simulink model "SecRwRtStBkReclnIsPosChk"  (R2024b)
settings: Solver=FixedStepDiscrete  StartTime=0.0  StopTime=10.0  FixedStep=0.01  RelTol=1e-3
undefined symbols (not defined in the file or in its folder): KeSMSuSecRwStBackPosDelta_Val, KeSMSuSecRwStBackPosTolr_Val, KeSMSuVehicleModelConfig_Val
libraries: StIsPosChkLib x19, simulink x8
(part 1 of 2)
settings Model: Creator=sn2xws  LastModifiedBy=sn55gm
settings Model: ModifiedHistory=|
  | 2023.8.1 V2.0.0 CR421790 增加模式21-26
  | 2024.3.14
  | V2.3.0
  | Bug 813950 童锁Lock，Mode1_Easy Entry Mode 不应调用失败
  | 2024.5.7 V3.0.0 557 eze模式变更
  | 2024.7.8 V3.0.1 557模式流程V1.9
  | 2024.8.15 V3.0.2 智享模式需要计算目标位置，不能直接判断到位置，posalready赋值0
  | 2024.8.20 V3.0.3 MD32到位置不看二排靠背
  | 2024.9.5 V3.0.4 增加Md56，注释掉不用的模式
  | 2024.10.14 V3.0.5 增加Md57，Md58
  | 2024.10.29 V3.0.6 6s版本不使用md8目标位置
  | 2024.11.5 V3.0.7 6s版本不动Md32
  | 2024.11.27 V3.0.8 Md57 运行时二排不能直接判断到位置
  | 2024.12.18 V3.0.8 md53 到位置不应看二排靠背，md32，md53同时动时，应用较小目标位置
  | 25.5.20 V3.12.0 童锁Md56应报成功
  | 25.7.1 V3.13.0 新增Md61 Md62
settings SolverCC: AlgebraicLoopSolver=TrustRegion
settings DataIOCC: SaveFormat=StructureWithTime  ReturnWorkspaceOutputs=off
settings OptimizationCC: DefaultParameterBehavior=Inlined  EnhancedBackFolding=on  PassReuseOutputArgsAs=Individual arguments  ZeroExternalMemoryAtStartup=off  ZeroInternalMemoryAtStartup=off  OptimizeBlockOrder=speed  DifferentSizesBufferReuse=on  OptimizationCustomize=off  EfficientTunableParamExpr=on
settings DebuggingCC: ParameterTunabilityLossMsg=error  UnconnectedInputMsg=warning  UnconnectedOutputMsg=warning  UnconnectedLineMsg=warning  ArithmeticOperatorsInVariantConditions=warning
settings ModelReferenceCC: EnableRefExpFcnMdlSchedulingChecks=on  ModelReferenceNumInstancesAllowed=Single
settings SFSimCC: MATLABDynamicMemAlloc=off  CustomCodeUndefinedFunction=UseInterfaceOnly
settings RTWCC: Description=AUTOSAR  SystemTargetFile=autosar.tlc  GenCodeOnly=on  TemplateMakefile=ert_default_tmf  GenerateReport=on  IncludeHyperlinkInReport=on  LaunchReport=on  DataTypeReplacement=CDataTypesFixedWidth  GenerateTraceInfo=on  GenerateTraceReport=on  GenerateTraceReportSl=on  GenerateTraceReportSf=on  GenerateTraceReportEml=on  GPUComputeCapability=3.5
settings CodeAppCC: ForceParamTrailComments=on  IgnoreCustomStorageClasses=off  OperatorAnnotations=on  SimulinkDataObjDesc=on  SFDataObjDesc=on  InsertBlockDesc=on
settings STFCustomTargetCC: TargetLangStandard=C99 (ISO)  MultiwordLength=256  ParMdlRefBuildCompliant=on  CompOptLevelCompliant=on  IncludeMdlTerminateFcn=off  CombineOutputUpdateFcns=on  SuppressErrorStatus=on  ERTCustomFileBanners=on  SupportNonFinite=off  SupportComplex=off  SupportContinuousTime=off  SupportNonInlinedSFcns=off  RemoveResetFunc=on  MATLABClassNameForMDSCustomization=Simulink.SoftwareTarget.ERTCustomization  AutosarCompliant=on  UseToolchainInfoCompliant=on  LookupTableObjectStructAxisOrder=2,1,3,4,...  LUTObjectStructOrderEvenSpacing=Size,Table,Breakpoints  SystemTargetFile=autosar.tlc
settings ERTTargetCC: TargetLangStandard=C99 (ISO)  ConcurrentExecutionCompliant=off  IncludeMdlTerminateFcn=off  SuppressErrorStatus=on  SupportNonFinite=off  SupportComplex=off  ModelStepFunctionPrototypeControlCompliant=off  CPPClassGenCompliant=off  AutosarCompliant=on  LookupTableObjectStructAxisOrder=2,1,3,4,...  LUTObjectStructOrderEvenSpacing=Size,Table,Breakpoints  ERTCustomFileTemplate=example_file_process.tlc  ERTFilePackagingFormat=Compact  BooleanTrueId=TRUE  BooleanFalseId=FALSE  DynamicArrayContainerType=coder::array

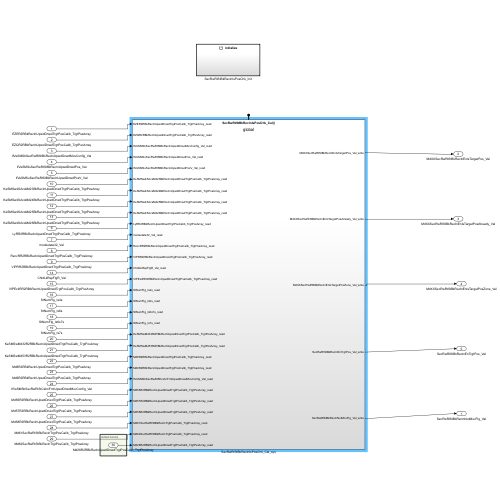
[thumbnail: Simulink's stored preview of the top-level diagram]
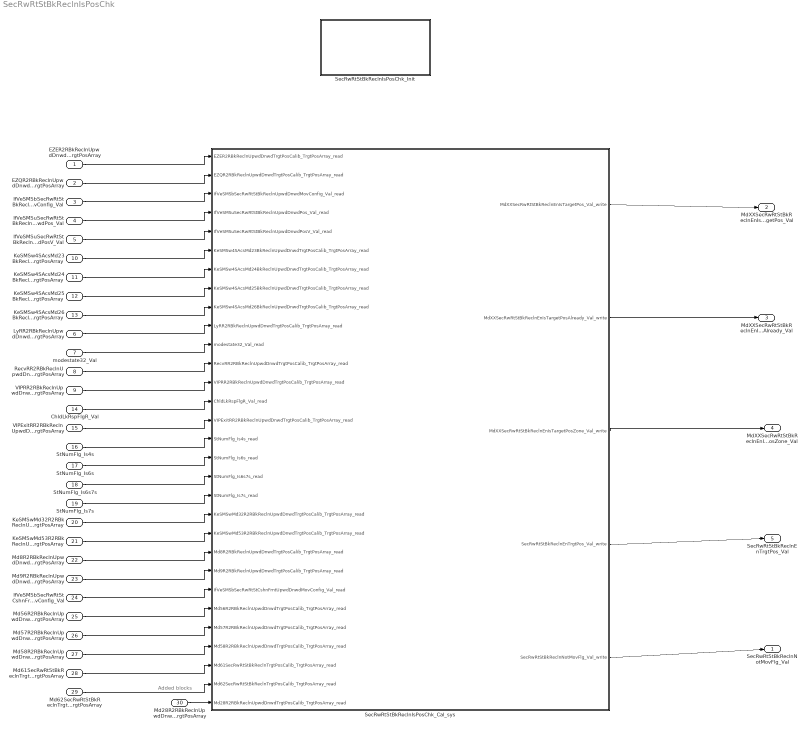
== system SecRwRtStBkReclnIsPosChk ==
  note: Added blocks
  EZER2RBkReclnUpwdDnwdTrgtPosCalib_TrgtPosArray : Inport  Description=|  OutDataTypeStr=uint16  PortDimensions=3
      | 0:Pos
      | 1:Max
      | 2:Min
  EZQR2RBkReclnUpwdDnwdTrgtPosCalib_TrgtPosArray : Inport  Description=|  Port=2  OutDataTypeStr=uint16  PortDimensions=3
      | 0:Pos
      | 1:Max
      | 2:Min
  IfVeSMSbSecRwRtStBkReclnUpwdDnwdMovConfig_Val : Inport  Port=3  OutDataTypeStr=boolean  PortDimensions=1
  IfVeSMSuSecRwRtStBkReclnUpwdDnwdPos_Val : Inport  Port=4  OutDataTypeStr=uint16  PortDimensions=1
  IfVeSMSuSecRwRtStBkReclnUpwdDnwdPosV_Val : Inport  Port=5  OutDataTypeStr=boolean  PortDimensions=1
  LyRR2RBkReclnUpwdDnwdTrgtPosCalib_TrgtPosArray : Inport  Description=|  Port=6  OutDataTypeStr=uint16  PortDimensions=3
      | 0:Pos
      | 1:Max
      | 2:Min
  modestate32_Val : Inport  Port=7  OutDataTypeStr=uint32  PortDimensions=1
  RecvRR2RBkReclnUpwdDnwdTrgtPosCalib_TrgtPosArray : Inport  Description=|  Port=8  OutDataTypeStr=uint16  PortDimensions=3
      | 0:Pos
      | 1:Max
      | 2:Min
  VIPRR2RBkReclnUpwdDnwdTrgtPosCalib_TrgtPosArray : Inport  Description=|  Port=9  OutDataTypeStr=uint16  PortDimensions=3
      | 0:Pos
      | 1:Max
      | 2:Min
  KeSMSw4SAcsMd23BkReclnUpwdDnwdTrgtPosCalib_TrgtPosArray : Inport  Description=|  Port=10  OutDataTypeStr=uint16  PortDimensions=3
      | 0:Pos
      | 1:Max
      | 2:Min
  KeSMSw4SAcsMd24BkReclnUpwdDnwdTrgtPosCalib_TrgtPosArray : Inport  Description=|  Port=11  OutDataTypeStr=uint16  PortDimensions=3
      | 0:Pos
      | 1:Max
      | 2:Min
  KeSMSw4SAcsMd25BkReclnUpwdDnwdTrgtPosCalib_TrgtPosArray : Inport  Description=|  Port=12  OutDataTypeStr=uint16  PortDimensions=3
      | 0:Pos
      | 1:Max
      | 2:Min
  KeSMSw4SAcsMd26BkReclnUpwdDnwdTrgtPosCalib_TrgtPosArray : Inport  Description=|  Port=13  OutDataTypeStr=uint16  PortDimensions=3
      | 0:Pos
      | 1:Max
      | 2:Min
  ChldLkRspFlgR_Val : Inport  Port=14  OutDataTypeStr=boolean  PortDimensions=1
  VIPExitRR2RBkReclnUpwdDnwdTrgtPosCalib_TrgtPosArray : Inport  Description=|  Port=15  OutDataTypeStr=uint16  PortDimensions=3
      | 0:Pos
      | 1:Max
      | 2:Min
  StNumFlg_Is4s : Inport  Port=16  OutDataTypeStr=boolean  PortDimensions=1
  StNumFlg_Is6s : Inport  Port=17  OutDataTypeStr=boolean  PortDimensions=1
  StNumFlg_Is6s7s : Inport  Port=18  OutDataTypeStr=boolean  PortDimensions=1
  StNumFlg_Is7s : Inport  Port=19  OutDataTypeStr=boolean  PortDimensions=1
  KeSMSwMd32R2RBkReclnUpwdDnwdTrgtPosCalib_TrgtPosArray : Inport  Description=|  Port=20  OutDataTypeStr=uint16  PortDimensions=3
      | 0:Pos
      | 1:Max
      | 2:Min
  KeSMSwMd53R2RBkReclnUpwdDnwdTrgtPosCalib_TrgtPosArray : Inport  Description=|  Port=21  OutDataTypeStr=uint16  PortDimensions=3
      | 0:Pos
      | 1:Max
      | 2:Min
  Md8R2RBkReclnUpwdDnwdTrgtPosCalib_TrgtPosArray : Inport  Description=|  Port=22  OutDataTypeStr=uint16  PortDimensions=3
      | 0:Pos
      | 1:Max
      | 2:Min
  Md9R2RBkReclnUpwdDnwdTrgtPosCalib_TrgtPosArray : Inport  Description=|  Port=23  OutDataTypeStr=uint16  PortDimensions=3
      | 0:Pos
      | 1:Max
      | 2:Min
  IfVeSMSbSecRwRtStCshnFrntUpwdDnwdMovConfig_Val : Inport  Port=24  OutDataTypeStr=boolean  PortDimensions=1
  Md56R2RBkReclnUpwdDnwdTrgtPosCalib_TrgtPosArray : Inport  Description=|  Port=25  OutDataTypeStr=uint16  PortDimensions=3
      | 0:Pos
      | 1:Max
      | 2:Min
  Md57R2RBkReclnUpwdDnwdTrgtPosCalib_TrgtPosArray : Inport  Description=|  Port=26  OutDataTypeStr=uint16  PortDimensions=3
      | 0:Pos
      | 1:Max
      | 2:Min
  Md58R2RBkReclnUpwdDnwdTrgtPosCalib_TrgtPosArray : Inport  Description=|  Port=27  OutDataTypeStr=uint16  PortDimensions=3
      | 0:Pos
      | 1:Max
      | 2:Min
  Md61SecRwRtStBkReclnTrgtPosCalib_TrgtPosArray : Inport  Description=|  Port=28  OutDataTypeStr=uint16  PortDimensions=3
      | 0:Pos
      | 1:Max
      | 2:Min
  Md62SecRwRtStBkReclnTrgtPosCalib_TrgtPosArray : Inport  Description=|  Port=29  OutDataTypeStr=uint16  PortDimensions=3
      | 0:Pos
      | 1:Max
      | 2:Min
  Md28R2RBkReclnUpwdDnwdTrgtPosCalib_TrgtPosArray : Inport  Description=|  Port=30  OutDataTypeStr=uint16  PortDimensions=3
      | 0:Pos
      | 1:Max
      | 2:Min
  SecRwRtStBkReclnIsPosChk_Cal_sys : Subsystem
  SecRwRtStBkReclnIsPosChk_Init : Subsystem
  SecRwRtStBkReclnNotMovFlg_Val : Outport  OutDataTypeStr=boolean  PortDimensions=1  VectorParamsAs1DForOutWhenUnconnected=off
  MdXXSecRwRtStBkReclnEnIsTargetPos_Val : Outport  Port=2  OutDataTypeStr=uint32  PortDimensions=1  VectorParamsAs1DForOutWhenUnconnected=off
  MdXXSecRwRtStBkReclnEnIsTargetPosAlready_Val : Outport  Port=3  OutDataTypeStr=uint32  PortDimensions=1  VectorParamsAs1DForOutWhenUnconnected=off
  MdXXSecRwRtStBkReclnEnIsTargetPosZone_Val : Outport  Port=4  OutDataTypeStr=uint32  PortDimensions=1  VectorParamsAs1DForOutWhenUnconnected=off
  SecRwRtStBkReclnEnTrgtPos_Val : Outport  Port=5  OutDataTypeStr=uint16  PortDimensions=1  VectorParamsAs1DForOutWhenUnconnected=off
  wires:
  EZER2RBkReclnUpwdDnwdTrgtPosCalib_TrgtPosArray/1 -> SecRwRtStBkReclnIsPosChk_Cal_sys/1(EZER2RBkReclnUpwdDnwdTrgtPosCalib_TrgtPosArray_read)
  EZQR2RBkReclnUpwdDnwdTrgtPosCalib_TrgtPosArray/1 -> SecRwRtStBkReclnIsPosChk_Cal_sys/2(EZQR2RBkReclnUpwdDnwdTrgtPosCalib_TrgtPosArray_read)
  IfVeSMSbSecRwRtStBkReclnUpwdDnwdMovConfig_Val/1 -> SecRwRtStBkReclnIsPosChk_Cal_sys/3(IfVeSMSbSecRwRtStBkReclnUpwdDnwdMovConfig_Val_read)
  IfVeSMSuSecRwRtStBkReclnUpwdDnwdPos_Val/1 -> SecRwRtStBkReclnIsPosChk_Cal_sys/4(IfVeSMSuSecRwRtStBkReclnUpwdDnwdPos_Val_read)
  IfVeSMSuSecRwRtStBkReclnUpwdDnwdPosV_Val/1 -> SecRwRtStBkReclnIsPosChk_Cal_sys/5(IfVeSMSuSecRwRtStBkReclnUpwdDnwdPosV_Val_read)
  LyRR2RBkReclnUpwdDnwdTrgtPosCalib_TrgtPosArray/1 -> SecRwRtStBkReclnIsPosChk_Cal_sys/10(LyRR2RBkReclnUpwdDnwdTrgtPosCalib_TrgtPosArray_read)
  modestate32_Val/1 -> SecRwRtStBkReclnIsPosChk_Cal_sys/11(modestate32_Val_read)
  RecvRR2RBkReclnUpwdDnwdTrgtPosCalib_TrgtPosArray/1 -> SecRwRtStBkReclnIsPosChk_Cal_sys/12(RecvRR2RBkReclnUpwdDnwdTrgtPosCalib_TrgtPosArray_read)
  VIPRR2RBkReclnUpwdDnwdTrgtPosCalib_TrgtPosArray/1 -> SecRwRtStBkReclnIsPosChk_Cal_sys/13(VIPRR2RBkReclnUpwdDnwdTrgtPosCalib_TrgtPosArray_read)
  SecRwRtStBkReclnIsPosChk_Cal_sys/1(MdXXSecRwRtStBkReclnEnIsTargetPos_Val_write) -> MdXXSecRwRtStBkReclnEnIsTargetPos_Val/1
  SecRwRtStBkReclnIsPosChk_Cal_sys/2(MdXXSecRwRtStBkReclnEnIsTargetPosAlready_Val_write) -> MdXXSecRwRtStBkReclnEnIsTargetPosAlready_Val/1
  SecRwRtStBkReclnIsPosChk_Cal_sys/3(MdXXSecRwRtStBkReclnEnIsTargetPosZone_Val_write) -> MdXXSecRwRtStBkReclnEnIsTargetPosZone_Val/1
  SecRwRtStBkReclnIsPosChk_Cal_sys/4(SecRwRtStBkReclnEnTrgtPos_Val_write) -> SecRwRtStBkReclnEnTrgtPos_Val/1
  SecRwRtStBkReclnIsPosChk_Cal_sys/5(SecRwRtStBkReclnNotMovFlg_Val_write) -> SecRwRtStBkReclnNotMovFlg_Val/1
  KeSMSw4SAcsMd23BkReclnUpwdDnwdTrgtPosCalib_TrgtPosArray/1 -> SecRwRtStBkReclnIsPosChk_Cal_sys/6(KeSMSw4SAcsMd23BkReclnUpwdDnwdTrgtPosCalib_TrgtPosArray_read)
  KeSMSw4SAcsMd24BkReclnUpwdDnwdTrgtPosCalib_TrgtPosArray/1 -> SecRwRtStBkReclnIsPosChk_Cal_sys/7(KeSMSw4SAcsMd24BkReclnUpwdDnwdTrgtPosCalib_TrgtPosArray_read)
  KeSMSw4SAcsMd25BkReclnUpwdDnwdTrgtPosCalib_TrgtPosArray/1 -> SecRwRtStBkReclnIsPosChk_Cal_sys/8(KeSMSw4SAcsMd25BkReclnUpwdDnwdTrgtPosCalib_TrgtPosArray_read)
  KeSMSw4SAcsMd26BkReclnUpwdDnwdTrgtPosCalib_TrgtPosArray/1 -> SecRwRtStBkReclnIsPosChk_Cal_sys/9(KeSMSw4SAcsMd26BkReclnUpwdDnwdTrgtPosCalib_TrgtPosArray_read)
  ChldLkRspFlgR_Val/1 -> SecRwRtStBkReclnIsPosChk_Cal_sys/14(ChldLkRspFlgR_Val_read)
  VIPExitRR2RBkReclnUpwdDnwdTrgtPosCalib_TrgtPosArray/1 -> SecRwRtStBkReclnIsPosChk_Cal_sys/15(VIPExitRR2RBkReclnUpwdDnwdTrgtPosCalib_TrgtPosArray_read)
  StNumFlg_Is4s/1 -> SecRwRtStBkReclnIsPosChk_Cal_sys/16(StNumFlg_Is4s_read)
  StNumFlg_Is6s/1 -> SecRwRtStBkReclnIsPosChk_Cal_sys/17(StNumFlg_Is6s_read)
  StNumFlg_Is6s7s/1 -> SecRwRtStBkReclnIsPosChk_Cal_sys/18(StNumFlg_Is6s7s_read)
  StNumFlg_Is7s/1 -> SecRwRtStBkReclnIsPosChk_Cal_sys/19(StNumFlg_Is7s_read)
  KeSMSwMd32R2RBkReclnUpwdDnwdTrgtPosCalib_TrgtPosArray/1 -> SecRwRtStBkReclnIsPosChk_Cal_sys/20(KeSMSwMd32R2RBkReclnUpwdDnwdTrgtPosCalib_TrgtPosArray_read)
  KeSMSwMd53R2RBkReclnUpwdDnwdTrgtPosCalib_TrgtPosArray/1 -> SecRwRtStBkReclnIsPosChk_Cal_sys/21(KeSMSwMd53R2RBkReclnUpwdDnwdTrgtPosCalib_TrgtPosArray_read)
  Md8R2RBkReclnUpwdDnwdTrgtPosCalib_TrgtPosArray/1 -> SecRwRtStBkReclnIsPosChk_Cal_sys/22(Md8R2RBkReclnUpwdDnwdTrgtPosCalib_TrgtPosArray_read)
  Md9R2RBkReclnUpwdDnwdTrgtPosCalib_TrgtPosArray/1 -> SecRwRtStBkReclnIsPosChk_Cal_sys/23(Md9R2RBkReclnUpwdDnwdTrgtPosCalib_TrgtPosArray_read)
  IfVeSMSbSecRwRtStCshnFrntUpwdDnwdMovConfig_Val/1 -> SecRwRtStBkReclnIsPosChk_Cal_sys/24(IfVeSMSbSecRwRtStCshnFrntUpwdDnwdMovConfig_Val_read)
  Md56R2RBkReclnUpwdDnwdTrgtPosCalib_TrgtPosArray/1 -> SecRwRtStBkReclnIsPosChk_Cal_sys/25(Md56R2RBkReclnUpwdDnwdTrgtPosCalib_TrgtPosArray_read)
  Md57R2RBkReclnUpwdDnwdTrgtPosCalib_TrgtPosArray/1 -> SecRwRtStBkReclnIsPosChk_Cal_sys/26(Md57R2RBkReclnUpwdDnwdTrgtPosCalib_TrgtPosArray_read)
  Md58R2RBkReclnUpwdDnwdTrgtPosCalib_TrgtPosArray/1 -> SecRwRtStBkReclnIsPosChk_Cal_sys/27(Md58R2RBkReclnUpwdDnwdTrgtPosCalib_TrgtPosArray_read)
  Md61SecRwRtStBkReclnTrgtPosCalib_TrgtPosArray/1 -> SecRwRtStBkReclnIsPosChk_Cal_sys/28(Md61SecRwRtStBkReclnTrgtPosCalib_TrgtPosArray_read)
  Md62SecRwRtStBkReclnTrgtPosCalib_TrgtPosArray/1 -> SecRwRtStBkReclnIsPosChk_Cal_sys/29(Md62SecRwRtStBkReclnTrgtPosCalib_TrgtPosArray_read)
  Md28R2RBkReclnUpwdDnwdTrgtPosCalib_TrgtPosArray/1 -> SecRwRtStBkReclnIsPosChk_Cal_sys/30(Md28R2RBkReclnUpwdDnwdTrgtPosCalib_TrgtPosArray_read)

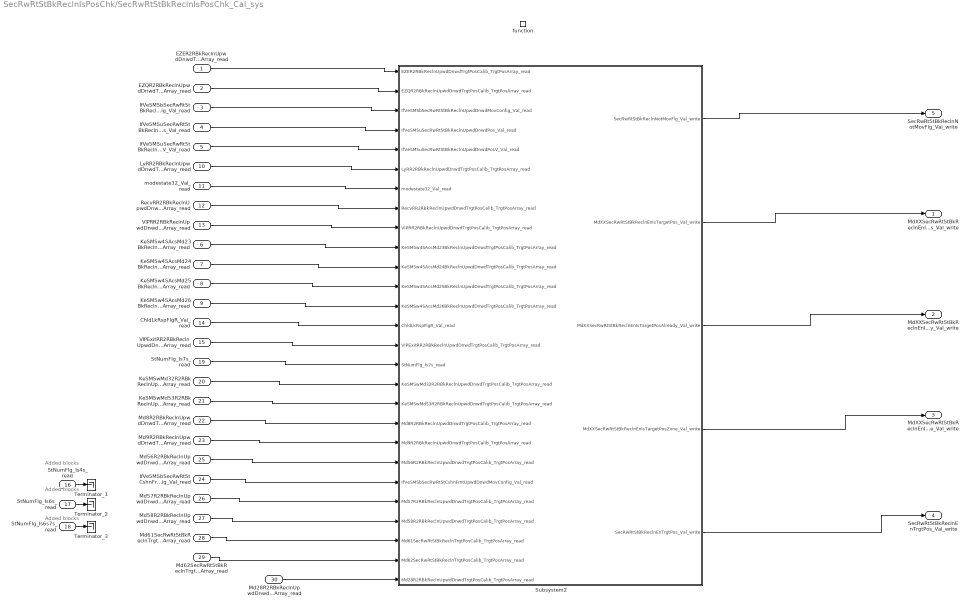
== system SecRwRtStBkReclnIsPosChk/SecRwRtStBkReclnIsPosChk_Cal_sys ==
  note: Added blocks
  note: Added blocks
  note: Added blocks
  EZER2RBkReclnUpwdDnwdTrgtPosCalib_TrgtPosArray_read : Inport
  EZQR2RBkReclnUpwdDnwdTrgtPosCalib_TrgtPosArray_read : Inport  Port=2
  IfVeSMSbSecRwRtStBkReclnUpwdDnwdMovConfig_Val_read : Inport  Port=3
  IfVeSMSuSecRwRtStBkReclnUpwdDnwdPos_Val_read : Inport  Port=4
  IfVeSMSuSecRwRtStBkReclnUpwdDnwdPosV_Val_read : Inport  Port=5
  KeSMSw4SAcsMd23BkReclnUpwdDnwdTrgtPosCalib_TrgtPosArray_read : Inport  Port=6
  KeSMSw4SAcsMd24BkReclnUpwdDnwdTrgtPosCalib_TrgtPosArray_read : Inport  Port=7
  KeSMSw4SAcsMd25BkReclnUpwdDnwdTrgtPosCalib_TrgtPosArray_read : Inport  Port=8
  KeSMSw4SAcsMd26BkReclnUpwdDnwdTrgtPosCalib_TrgtPosArray_read : Inport  Port=9
  LyRR2RBkReclnUpwdDnwdTrgtPosCalib_TrgtPosArray_read : Inport  Port=10
  modestate32_Val_read : Inport  Port=11
  RecvRR2RBkReclnUpwdDnwdTrgtPosCalib_TrgtPosArray_read : Inport  Port=12
  VIPRR2RBkReclnUpwdDnwdTrgtPosCalib_TrgtPosArray_read : Inport  Port=13
  ChldLkRspFlgR_Val_read : Inport  Port=14
  VIPExitRR2RBkReclnUpwdDnwdTrgtPosCalib_TrgtPosArray_read : Inport  Port=15
  StNumFlg_Is4s_read : Inport  Port=16
  StNumFlg_Is6s_read : Inport  Port=17
  StNumFlg_Is6s7s_read : Inport  Port=18
  StNumFlg_Is7s_read : Inport  Port=19
  KeSMSwMd32R2RBkReclnUpwdDnwdTrgtPosCalib_TrgtPosArray_read : Inport  Port=20
  KeSMSwMd53R2RBkReclnUpwdDnwdTrgtPosCalib_TrgtPosArray_read : Inport  Port=21
  Md8R2RBkReclnUpwdDnwdTrgtPosCalib_TrgtPosArray_read : Inport  Port=22
  Md9R2RBkReclnUpwdDnwdTrgtPosCalib_TrgtPosArray_read : Inport  Port=23
  IfVeSMSbSecRwRtStCshnFrntUpwdDnwdMovConfig_Val_read : Inport  Port=24
  Md56R2RBkReclnUpwdDnwdTrgtPosCalib_TrgtPosArray_read : Inport  Port=25
  Md57R2RBkReclnUpwdDnwdTrgtPosCalib_TrgtPosArray_read : Inport  Port=26
  Md58R2RBkReclnUpwdDnwdTrgtPosCalib_TrgtPosArray_read : Inport  Port=27
  Md61SecRwRtStBkReclnTrgtPosCalib_TrgtPosArray_read : Inport  Port=28
  Md62SecRwRtStBkReclnTrgtPosCalib_TrgtPosArray_read : Inport  Port=29
  Md28R2RBkReclnUpwdDnwdTrgtPosCalib_TrgtPosArray_read : Inport  Port=30
  function : TriggerPort  TriggerType=function-call  IsSimulinkFunction=on  FunctionName=SecRwRtStBkReclnIsPosChk_Cal  VariantControl=(inherit)
  Subsystem2 : Subsystem
  Terminator_1 : Terminator
  Terminator_2 : Terminator
  Terminator_3 : Terminator
  MdXXSecRwRtStBkReclnEnIsTargetPos_Val_write : Outport  VectorParamsAs1DForOutWhenUnconnected=off
      settings: EnsureOutportIsVirtual=on
  MdXXSecRwRtStBkReclnEnIsTargetPosAlready_Val_write : Outport  Port=2  VectorParamsAs1DForOutWhenUnconnected=off
      settings: EnsureOutportIsVirtual=on
  MdXXSecRwRtStBkReclnEnIsTargetPosZone_Val_write : Outport  Port=3  VectorParamsAs1DForOutWhenUnconnected=off
      settings: EnsureOutportIsVirtual=on
  SecRwRtStBkReclnEnTrgtPos_Val_write : Outport  Port=4  VectorParamsAs1DForOutWhenUnconnected=off
      settings: EnsureOutportIsVirtual=on
  SecRwRtStBkReclnNotMovFlg_Val_write : Outport  Port=5  VectorParamsAs1DForOutWhenUnconnected=off
      settings: EnsureOutportIsVirtual=on
  wires:
  LyRR2RBkReclnUpwdDnwdTrgtPosCalib_TrgtPosArray_read/1 -> Subsystem2/6(LyRR2RBkReclnUpwdDnwdTrgtPosCalib_TrgtPosArray_read)
  modestate32_Val_read/1 -> Subsystem2/7(modestate32_Val_read)
  RecvRR2RBkReclnUpwdDnwdTrgtPosCalib_TrgtPosArray_read/1 -> Subsystem2/8(RecvRR2RBkReclnUpwdDnwdTrgtPosCalib_TrgtPosArray_read)
  IfVeSMSuSecRwRtStBkReclnUpwdDnwdPosV_Val_read/1 -> Subsystem2/5(IfVeSMSuSecRwRtStBkReclnUpwdDnwdPosV_Val_read)
  VIPRR2RBkReclnUpwdDnwdTrgtPosCalib_TrgtPosArray_read/1 -> Subsystem2/9(VIPRR2RBkReclnUpwdDnwdTrgtPosCalib_TrgtPosArray_read)
  IfVeSMSbSecRwRtStBkReclnUpwdDnwdMovConfig_Val_read/1 -> Subsystem2/3(IfVeSMSbSecRwRtStBkReclnUpwdDnwdMovConfig_Val_read)
  IfVeSMSuSecRwRtStBkReclnUpwdDnwdPos_Val_read/1 -> Subsystem2/4(IfVeSMSuSecRwRtStBkReclnUpwdDnwdPos_Val_read)
  KeSMSw4SAcsMd23BkReclnUpwdDnwdTrgtPosCalib_TrgtPosArray_read/1 -> Subsystem2/10(KeSMSw4SAcsMd23BkReclnUpwdDnwdTrgtPosCalib_TrgtPosArray_read)
  EZQR2RBkReclnUpwdDnwdTrgtPosCalib_TrgtPosArray_read/1 -> Subsystem2/2(EZQR2RBkReclnUpwdDnwdTrgtPosCalib_TrgtPosArray_read)
  KeSMSw4SAcsMd24BkReclnUpwdDnwdTrgtPosCalib_TrgtPosArray_read/1 -> Subsystem2/11(KeSMSw4SAcsMd24BkReclnUpwdDnwdTrgtPosCalib_TrgtPosArray_read)
  EZER2RBkReclnUpwdDnwdTrgtPosCalib_TrgtPosArray_read/1 -> Subsystem2/1(EZER2RBkReclnUpwdDnwdTrgtPosCalib_TrgtPosArray_read)
  KeSMSw4SAcsMd25BkReclnUpwdDnwdTrgtPosCalib_TrgtPosArray_read/1 -> Subsystem2/12(KeSMSw4SAcsMd25BkReclnUpwdDnwdTrgtPosCalib_TrgtPosArray_read)
  KeSMSw4SAcsMd26BkReclnUpwdDnwdTrgtPosCalib_TrgtPosArray_read/1 -> Subsystem2/13(KeSMSw4SAcsMd26BkReclnUpwdDnwdTrgtPosCalib_TrgtPosArray_read)
  Subsystem2/1(SecRwRtStBkReclnNotMovFlg_Val_write) -> SecRwRtStBkReclnNotMovFlg_Val_write/1
  Subsystem2/2(MdXXSecRwRtStBkReclnEnIsTargetPos_Val_write) -> MdXXSecRwRtStBkReclnEnIsTargetPos_Val_write/1
  Subsystem2/3(MdXXSecRwRtStBkReclnEnIsTargetPosAlready_Val_write) -> MdXXSecRwRtStBkReclnEnIsTargetPosAlready_Val_write/1
  Subsystem2/4(MdXXSecRwRtStBkReclnEnIsTargetPosZone_Val_write) -> MdXXSecRwRtStBkReclnEnIsTargetPosZone_Val_write/1
  Subsystem2/5(SecRwRtStBkReclnEnTrgtPos_Val_write) -> SecRwRtStBkReclnEnTrgtPos_Val_write/1
  ChldLkRspFlgR_Val_read/1 -> Subsystem2/14(ChldLkRspFlgR_Val_read)
  VIPExitRR2RBkReclnUpwdDnwdTrgtPosCalib_TrgtPosArray_read/1 -> Subsystem2/15(VIPExitRR2RBkReclnUpwdDnwdTrgtPosCalib_TrgtPosArray_read)
  StNumFlg_Is4s_read/1 -> Terminator_1/1
  StNumFlg_Is6s_read/1 -> Terminator_2/1
  StNumFlg_Is6s7s_read/1 -> Terminator_3/1
  StNumFlg_Is7s_read/1 -> Subsystem2/16(StNumFlg_Is7s_read)
  KeSMSwMd32R2RBkReclnUpwdDnwdTrgtPosCalib_TrgtPosArray_read/1 -> Subsystem2/17(KeSMSwMd32R2RBkReclnUpwdDnwdTrgtPosCalib_TrgtPosArray_read)
  KeSMSwMd53R2RBkReclnUpwdDnwdTrgtPosCalib_TrgtPosArray_read/1 -> Subsystem2/18(KeSMSwMd53R2RBkReclnUpwdDnwdTrgtPosCalib_TrgtPosArray_read)
  Md8R2RBkReclnUpwdDnwdTrgtPosCalib_TrgtPosArray_read/1 -> Subsystem2/19(Md8R2RBkReclnUpwdDnwdTrgtPosCalib_TrgtPosArray_read)
  Md9R2RBkReclnUpwdDnwdTrgtPosCalib_TrgtPosArray_read/1 -> Subsystem2/20(Md9R2RBkReclnUpwdDnwdTrgtPosCalib_TrgtPosArray_read)
  Md56R2RBkReclnUpwdDnwdTrgtPosCalib_TrgtPosArray_read/1 -> Subsystem2/21(Md56R2RBkReclnUpwdDnwdTrgtPosCalib_TrgtPosArray_read)
  IfVeSMSbSecRwRtStCshnFrntUpwdDnwdMovConfig_Val_read/1 -> Subsystem2/22(IfVeSMSbSecRwRtStCshnFrntUpwdDnwdMovConfig_Val_read)
  Md57R2RBkReclnUpwdDnwdTrgtPosCalib_TrgtPosArray_read/1 -> Subsystem2/23(Md57R2RBkReclnUpwdDnwdTrgtPosCalib_TrgtPosArray_read)
  Md58R2RBkReclnUpwdDnwdTrgtPosCalib_TrgtPosArray_read/1 -> Subsystem2/24(Md58R2RBkReclnUpwdDnwdTrgtPosCalib_TrgtPosArray_read)
  Md61SecRwRtStBkReclnTrgtPosCalib_TrgtPosArray_read/1 -> Subsystem2/25(Md61SecRwRtStBkReclnTrgtPosCalib_TrgtPosArray_read)
  Md62SecRwRtStBkReclnTrgtPosCalib_TrgtPosArray_read/1 -> Subsystem2/26(Md62SecRwRtStBkReclnTrgtPosCalib_TrgtPosArray_read)
  Md28R2RBkReclnUpwdDnwdTrgtPosCalib_TrgtPosArray_read/1 -> Subsystem2/27(Md28R2RBkReclnUpwdDnwdTrgtPosCalib_TrgtPosArray_read)

== system SecRwRtStBkReclnIsPosChk/SecRwRtStBkReclnIsPosChk_Init ==
  note: Added blocks
  note: Added blocks
  note: Added blocks
  Event Listener : EventListener  EventName=reset
  PA_KeSMSuSecRwStBackPosDelta_Val : Constant  Value=KeSMSuSecRwStBackPosDelta_Val
  PA_KeSMSuSecRwStBackPosTolr_Val : Constant  Value=KeSMSuSecRwStBackPosTolr_Val
  PA_KeSMSuVehicleModelConfig_Val : Constant  Value=KeSMSuVehicleModelConfig_Val
  Terminator_1 : Terminator
  Terminator_2 : Terminator
  Terminator_3 : Terminator
  wires:
  PA_KeSMSuSecRwStBackPosDelta_Val/1 -> Terminator_1/1
  PA_KeSMSuSecRwStBackPosTolr_Val/1 -> Terminator_2/1
  PA_KeSMSuVehicleModelConfig_Val/1 -> Terminator_3/1

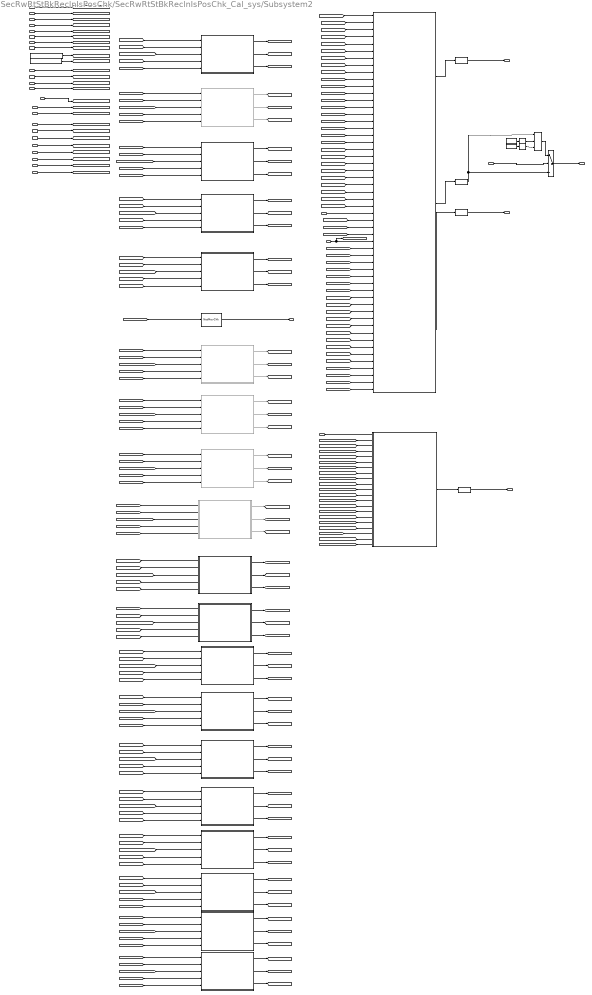
== system SecRwRtStBkReclnIsPosChk/SecRwRtStBkReclnIsPosChk_Cal_sys/Subsystem2 ==
  note: 2023.8.1 V2.0.0 CR421790 增加模式21-26
  EZER2RBkReclnUpwdDnwdTrgtPosCalib_TrgtPosArray_read : Inport
  EZQR2RBkReclnUpwdDnwdTrgtPosCalib_TrgtPosArray_read : Inport  Port=2
  IfVeSMSbSecRwRtStBkReclnUpwdDnwdMovConfig_Val_read : Inport  Port=3
  IfVeSMSuSecRwRtStBkReclnUpwdDnwdPos_Val_read : Inport  Port=4
  IfVeSMSuSecRwRtStBkReclnUpwdDnwdPosV_Val_read : Inport  Port=5
  LyRR2RBkReclnUpwdDnwdTrgtPosCalib_TrgtPosArray_read : Inport  Port=6
  modestate32_Val_read : Inport  Port=7
  RecvRR2RBkReclnUpwdDnwdTrgtPosCalib_TrgtPosArray_read : Inport  Port=8
  VIPRR2RBkReclnUpwdDnwdTrgtPosCalib_TrgtPosArray_read : Inport  Port=9
  KeSMSw4SAcsMd23BkReclnUpwdDnwdTrgtPosCalib_TrgtPosArray_read : Inport  Port=10
  KeSMSw4SAcsMd24BkReclnUpwdDnwdTrgtPosCalib_TrgtPosArray_read : Inport  Port=11
  KeSMSw4SAcsMd25BkReclnUpwdDnwdTrgtPosCalib_TrgtPosArray_read : Inport  Port=12
  KeSMSw4SAcsMd26BkReclnUpwdDnwdTrgtPosCalib_TrgtPosArray_read : Inport  Port=13
  ChldLkRspFlgR_Val_read : Inport  Port=14
  VIPExitRR2RBkReclnUpwdDnwdTrgtPosCalib_TrgtPosArray_read : Inport  Port=15
  StNumFlg_Is7s_read : Inport  Port=16
  KeSMSwMd32R2RBkReclnUpwdDnwdTrgtPosCalib_TrgtPosArray_read : Inport  Port=17
  KeSMSwMd53R2RBkReclnUpwdDnwdTrgtPosCalib_TrgtPosArray_read : Inport  Port=18
  Md8R2RBkReclnUpwdDnwdTrgtPosCalib_TrgtPosArray_read : Inport  Port=19
  Md9R2RBkReclnUpwdDnwdTrgtPosCalib_TrgtPosArray_read : Inport  Port=20
  Md56R2RBkReclnUpwdDnwdTrgtPosCalib_TrgtPosArray_read : Inport  Port=21
  IfVeSMSbSecRwRtStCshnFrntUpwdDnwdMovConfig_Val_read : Inport  Port=22
  Md57R2RBkReclnUpwdDnwdTrgtPosCalib_TrgtPosArray_read : Inport  Port=23
  Md58R2RBkReclnUpwdDnwdTrgtPosCalib_TrgtPosArray_read : Inport  Port=24
  Md61SecRwRtStBkReclnTrgtPosCalib_TrgtPosArray_read : Inport  Port=25
  Md62SecRwRtStBkReclnTrgtPosCalib_TrgtPosArray_read : Inport  Port=26
  Md28R2RBkReclnUpwdDnwdTrgtPosCalib_TrgtPosArray_read : Inport  Port=27
  Bitwise Operator : simulink/Logic and Bit Operations/Bitwise Operator  logicop=AND  UseBitMask=off  NumInputPorts=3  BitMask=bin2dec('11011001')  BitMaskRealWorld=Stored Integer
  Bitwise Operator1 : simulink/Logic and Bit Operations/Bitwise Operator  logicop=NOT  UseBitMask=off  BitMask=bin2dec('11011001')  BitMaskRealWorld=Stored Integer
  Bitwise Operator2 : simulink/Logic and Bit Operations/Bitwise Operator  logicop=NOT  UseBitMask=off  BitMask=bin2dec('11011001')  BitMaskRealWorld=Stored Integer
  Constant : Constant  Value=2048  OutDataTypeStr=uint32
  Constant1 : Constant  Value=1048576  OutDataTypeStr=uint32
  Data Type Conversion{,1..3} (4 alike) : DataTypeConversion  SaturateOnIntegerOverflow=off  RndMeth=Floor
  NotMovChk : StIsPosChkLib/NotMovChk  SystemSampleTime=-1  VariantActivationTime=update diagram  AllowFlexibleInterface=on  Latency=0  AutoFrameSizeCalculation=off
  PA_KeSMSuSecRwStBackPosDelta_Val : Constant  Value=KeSMSuSecRwStBackPosDelta_Val
  PA_KeSMSuSecRwStBackPosTolr_Val : Constant  Value=KeSMSuSecRwStBackPosTolr_Val
  Subsystem : Subsystem
  Subsystem1 : Subsystem
  Subsystem10 : Subsystem  Commented=on
  Subsystem11 : Subsystem
  Subsystem12 : Subsystem
  Subsystem13 : Subsystem
  Subsystem14 : Subsystem
  Subsystem15 : Subsystem
  Subsystem16 : Subsystem
  Subsystem17 : Subsystem
  Subsystem18 : Subsystem
  Subsystem19 : Subsystem
  Subsystem2 : Subsystem
  Subsystem20 : Subsystem
  Subsystem3 : Subsystem  Commented=on
  Subsystem4 : Subsystem
  Subsystem5 : Subsystem
  Subsystem6 : Subsystem
  Subsystem7 : Subsystem  Commented=on
  Subsystem8 : Subsystem  Commented=on
  Subsystem9 : Subsystem  Commented=on
  Switch : Switch  Criteria=u2 > Threshold  SaturateOnIntegerOverflow=off  InputSameDT=off
  SecRwRtStBkReclnNotMovFlg_Val_write : Outport  VectorParamsAs1DForOutWhenUnconnected=off
      settings: EnsureOutportIsVirtual=on
  MdXXSecRwRtStBkReclnEnIsTargetPos_Val_write : Outport  Port=2  VectorParamsAs1DForOutWhenUnconnected=off
      settings: EnsureOutportIsVirtual=on
  MdXXSecRwRtStBkReclnEnIsTargetPosAlready_Val_write : Outport  Port=3  VectorParamsAs1DForOutWhenUnconnected=off
      settings: EnsureOutportIsVirtual=on
  MdXXSecRwRtStBkReclnEnIsTargetPosZone_Val_write : Outport  Port=4  VectorParamsAs1DForOutWhenUnconnected=off
      settings: EnsureOutportIsVirtual=on
  SecRwRtStBkReclnEnTrgtPos_Val_write : Outport  Port=5  VectorParamsAs1DForOutWhenUnconnected=off
      settings: EnsureOutportIsVirtual=on
  wires:
  Data Type Conversion1/1 -> MdXXSecRwRtStBkReclnEnIsTargetPosZone_Val_write/1
  [EZQCalib] -> Subsystem3/3(CalibArray)
  [VIPRCalib] -> Subsystem6/3(CalibArray)
  [PosTolr] -> Subsystem5/5(Tolr)
  [PosDelta] -> Subsystem2/4(Delta)
  [RecvLIsTargetPosZone] -> Subsystem1/15(RecvLIsTargetPosZone)
  [PosDelta] -> Subsystem3/4(Delta)
  Subsystem1/3(IsTargetPosZone) -> Data Type Conversion1/1
  [PosDelta] -> Subsystem4/4(Delta)
  [Pos] -> Subsystem3/2(Pos)
  Subsystem2/2(IsPosZone) -> [EZEIsTargetPosZone]
  Subsystem/1(TrgtPos) -> Data Type Conversion/1
  Subsystem2/1(IsPos) -> [EZEIsTargetPos]
  [PosDelta] -> Subsystem5/4(Delta)
  [PosTolr] -> Subsystem6/5(Tolr)
  [EZEIsTargetPos] -> Subsystem1/2(EZEIsTargetPos)
  Subsystem1/2(IsTargetPosAlready) -> Data Type Conversion2/1
  [EZQIsTargetPos] -> Subsystem1/3(EZQIsTargetPos)
  [PosTolr] -> Subsystem3/5(Tolr)
  [PosV] -> Subsystem6/1(PosV)
  NotMovChk/1 -> SecRwRtStBkReclnNotMovFlg_Val_write/1
  [EZECalib] -> Subsystem2/3(CalibArray)
  [EZQIsTargetPosZone] -> Subsystem1/13(EZQIsTargetPosZone)
  Subsystem1/1(IsTargetPos) -> Data Type Conversion3/1
  [Pos] -> Subsystem2/2(Pos)
  PA_KeSMSuSecRwStBackPosTolr_Val/1 -> [PosTolr]
  EZER2RBkReclnUpwdDnwdTrgtPosCalib_TrgtPosArray_read/1 -> [EZECalib]
  [Pos] -> Subsystem5/2(Pos)
  [Pos] -> NotMovChk/1
  Data Type Conversion/1 -> SecRwRtStBkReclnEnTrgtPos_Val_write/1
  [VIPRCalib] -> Subsystem/6(VIPLCalib)
  Subsystem3/1(IsPos) -> [EZQIsTargetPos]
  [MovConfig] -> Subsystem1/1(MovConfig)
  Subsystem6/2(IsPosZone) -> [VIPLIsTargetPosZone]
  Subsystem6/1(IsPos) -> [VIPLIsTargetPos]
  [VIPLIsTargetPosAlready] -> Subsystem1/11(VIPRIsTargetPosAlready)
  [EZEIsTargetPosAlready] -> Subsystem1/7(EZEIsTargetPosAlready)
  Subsystem4/3(IsPosAlready) -> [LyLIsTargetPosAlready]
  VIPRR2RBkReclnUpwdDnwdTrgtPosCalib_TrgtPosArray_read/1 -> [VIPRCalib]
  Subsystem4/2(IsPosZone) -> [LyLIsTargetPosZone]
  [RecvLIsTargetPos] -> Subsystem1/5(RecvLIsTargetPos)
  [PosV] -> Subsystem4/1(PosV)
  [RecvLIsTargetPosAlready] -> Subsystem1/10(RecvRIsTargetPosAlready)
  [PosTolr] -> Subsystem2/5(Tolr)
  Data Type Conversion3/1 -> MdXXSecRwRtStBkReclnEnIsTargetPos_Val_write/1
  [EZQCalib] -> Subsystem/3(EZQCalib)
  Subsystem2/3(IsPosAlready) -> [EZEIsTargetPosAlready]
  [EZQIsTargetPosAlready] -> Subsystem1/8(EZQIsTargetPosAlready)
  EZQR2RBkReclnUpwdDnwdTrgtPosCalib_TrgtPosArray_read/1 -> [EZQCalib]
  [EZECalib] -> Subsystem/2(EZECalib)
  IfVeSMSuSecRwRtStBkReclnUpwdDnwdPosV_Val_read/1 -> [PosV]
  [PosV] -> Subsystem5/1(PosV)
  PA_KeSMSuSecRwStBackPosDelta_Val/1 -> [PosDelta]
  [LyLIsTargetPosAlready] -> Subsystem1/9(LyRIsTargetPosAlready)
  Subsystem5/1(IsPos) -> [RecvLIsTargetPos]
  IfVeSMSuSecRwRtStBkReclnUpwdDnwdPos_Val_read/1 -> [Pos]
  LyRR2RBkReclnUpwdDnwdTrgtPosCalib_TrgtPosArray_read/1 -> [LyRCalib]
  [PosTolr] -> Subsystem4/5(Tolr)
  RecvRR2RBkReclnUpwdDnwdTrgtPosCalib_TrgtPosArray_read/1 -> [RecvRCalib]
  Subsystem6/3(IsPosAlready) -> [VIPLIsTargetPosAlready]
  Subsystem5/2(IsPosZone) -> [RecvLIsTargetPosZone]
  Subsystem3/3(IsPosAlready) -> [EZQIsTargetPosAlready]
  IfVeSMSbSecRwRtStBkReclnUpwdDnwdMovConfig_Val_read/1 -> [MovConfig]
  Subsystem4/1(IsPos) -> [LyLIsTargetPos]
  Subsystem3/2(IsPosZone) -> [EZQIsTargetPosZone]
  [PosV] -> Subsystem3/1(PosV)
  [Pos] -> Subsystem6/2(Pos)
  [PosV] -> Subsystem2/1(PosV)
  [RecvRCalib] -> Subsystem/5(RecvLCalib)
  [VIPLIsTargetPosZone] -> Subsystem1/16(VIPLIsTargetPosZone)
  [VIPLIsTargetPos] -> Subsystem1/6(VIPLIsTargetPos)
  [RecvRCalib] -> Subsystem5/3(CalibArray)
  [PosDelta] -> Subsystem6/4(Delta)
  [Md15Calib] -> Subsystem/4(LyLCalib)
  [LyLIsTargetPos] -> Subsystem1/4(LyLIsTargetPos)
  [LyLIsTargetPosZone] -> Subsystem1/14(LyLIsTargetPosZone)
  [Pos] -> Subsystem4/2(Pos)
  [Md15Calib] -> Subsystem4/3(CalibArray)
  [EZEIsTargetPosZone] -> Subsystem1/12(EZEIsTargetPosZone)
  modestate32_Val_read/1 -> Subsystem/1(modestate32_Val_read)
  Subsystem5/3(IsPosAlready) -> [RecvLIsTargetPosAlready]
  KeSMSw4SAcsMd23BkReclnUpwdDnwdTrgtPosCalib_TrgtPosArray_read/1 -> [Md23Calib]
  KeSMSw4SAcsMd26BkReclnUpwdDnwdTrgtPosCalib_TrgtPosArray_read/1 -> [Md26Calib]
  KeSMSw4SAcsMd25BkReclnUpwdDnwdTrgtPosCalib_TrgtPosArray_read/1 -> [Md25Calib]
  KeSMSw4SAcsMd24BkReclnUpwdDnwdTrgtPosCalib_TrgtPosArray_read/1 -> [Md24Calib]
  [PosTolr] -> Subsystem7/5(Tolr)
  [Md23Calib] -> Subsystem7/3(CalibArray)
  [Pos] -> Subsystem7/2(Pos)
  Subsystem7/3(IsPosAlready) -> [Md23IsTargetPosAlready]
  Subsystem7/1(IsPos) -> [Md23IsTargetPos]
  [PosV] -> Subsystem7/1(PosV)
  Subsystem7/2(IsPosZone) -> [Md23IsTargetPosZone]
  [PosDelta] -> Subsystem7/4(Delta)
  [PosDelta] -> Subsystem8/4(Delta)
  Subsystem8/2(IsPosZone) -> [Md24IsTargetPosZone]
  [PosV] -> Subsystem8/1(PosV)
  Subsystem8/1(IsPos) -> [Md24IsTargetPos]
  Subsystem8/3(IsPosAlready) -> [Md24IsTargetPosAlready]
  [Pos] -> Subsystem8/2(Pos)
  [Md24Calib] -> Subsystem8/3(CalibArray)
  [PosTolr] -> Subsystem8/5(Tolr)
  [PosTolr] -> Subsystem9/5(Tolr)
  [Md25Calib] -> Subsystem9/3(CalibArray)
  [Pos] -> Subsystem9/2(Pos)
  Subsystem9/3(IsPosAlready) -> [Md25IsTargetPosAlready]
  Subsystem9/1(IsPos) -> [Md25IsTargetPos]
  [PosV] -> Subsystem9/1(PosV)
  Subsystem9/2(IsPosZone) -> [Md25IsTargetPosZone]
  [PosDelta] -> Subsystem9/4(Delta)
  [PosDelta] -> Subsystem10/4(Delta)
  Subsystem10/2(IsPosZone) -> [Md26IsTargetPosZone]
  [PosV] -> Subsystem10/1(PosV)
  Subsystem10/1(IsPos) -> [Md26IsTargetPos]
  Subsystem10/3(IsPosAlready) -> [Md26IsTargetPosAlready]
  [Pos] -> Subsystem10/2(Pos)
  [Md26Calib] -> Subsystem10/3(CalibArray)
  [PosTolr] -> Subsystem10/5(Tolr)
  [Md23Calib] -> Subsystem/7(Md23Calib)
  [Md24Calib] -> Subsystem/8(Md24Calib)
  [Md25Calib] -> Subsystem/9(Md25Calib)
  [Md26Calib] -> Subsystem/10(Md26Calib)
  [Md23IsTargetPos] -> Subsystem1/17(Md23IsTargetPos)
  [Md24IsTargetPos] -> Subsystem1/18(Md24IsTargetPos)
  [Md57IsTargetPos] -> Subsystem1/19(Md57IsTargetPos)
  [Md58IsTargetPos] -> Subsystem1/20(Md58IsTargetPos)
  [Md23IsTargetPosAlready] -> Subsystem1/21(Md23IsTargetPosAlready)
  [Md24IsTargetPosAlready] -> Subsystem1/22(Md24IsTargetPosAlready)
  [Md57IsTargetPosAlready] -> Subsystem1/23(Md57IsTargetPosAlready)
  [Md58IsTargetPosAlready] -> Subsystem1/24(Md58IsTargetPosAlready)
  [Md23IsTargetPosZone] -> Subsystem1/25(Md23IsTargetPosZone)
  [Md24IsTargetPosZone] -> Subsystem1/26(Md24IsTargetPosZone)
  [Md57IsTargetPosZone] -> Subsystem1/27(Md57IsTargetPosZone)
  [Md58IsTargetPosZone] -> Subsystem1/28(Md58IsTargetPosZone)
  ChldLkRspFlgR_Val_read/1 -> Subsystem1/29(ChldLkRspFlgR_Val_read)
  [PosTolr] -> Subsystem11/5(Tolr)
  [Md28Calib] -> Subsystem11/3(CalibArray)
  [Pos] -> Subsystem11/2(Pos)
  Subsystem11/3(IsPosAlready) -> [Md28IsTargetPosAlready]
  Subsystem11/1(IsPos) -> [Md28IsTargetPos]
  [PosV] -> Subsystem11/1(PosV)
  Subsystem11/2(IsPosZone) -> [Md28IsTargetPosZone]
  [PosDelta] -> Subsystem11/4(Delta)
  [Md28Calib] -> Subsystem/11(Md28Calib)
  [Md28IsTargetPos] -> Subsystem1/30(Md28IsTargetPos)
  [Md28IsTargetPosAlready] -> Subsystem1/31(Md28IsTargetPosAlready)
  [Md28IsTargetPosZone] -> Subsystem1/32(Md28IsTargetPosZone)
  StNumFlg_Is7s_read/1 -> [is7s], Subsystem1/33(StNumFlg_Is7s_read)
  KeSMSwMd32R2RBkReclnUpwdDnwdTrgtPosCalib_TrgtPosArray_read/1 -> [Md32Calib]
  KeSMSwMd53R2RBkReclnUpwdDnwdTrgtPosCalib_TrgtPosArray_read/1 -> [Md53Calib]
  [PosDelta] -> Subsystem12/4(Delta)
  Subsystem12/2(IsPosZone) -> [Md32IsTargetPosZone]
  [PosV] -> Subsystem12/1(PosV)
  Subsystem12/1(IsPos) -> [Md32IsTargetPos]
  Subsystem12/3(IsPosAlready) -> [Md32IsTargetPosAlready]
  [Pos] -> Subsystem12/2(Pos)
  [Md32Calib] -> Subsystem12/3(CalibArray)
  [PosTolr] -> Subsystem12/5(Tolr)
  [PosTolr] -> Subsystem13/5(Tolr)
  [Md53Calib] -> Subsystem13/3(CalibArray)
  [Pos] -> Subsystem13/2(Pos)
  Subsystem13/3(IsPosAlready) -> [Md53IsTargetPosAlready]
  Subsystem13/1(IsPos) -> [Md53IsTargetPos]
  [PosV] -> Subsystem13/1(PosV)
  Subsystem13/2(IsPosZone) -> [Md53IsTargetPosZone]
  [PosDelta] -> Subsystem13/4(Delta)
  [Md32Calib] -> Subsystem/12(Md32Calib)
  [Md53Calib] -> Subsystem/13(Md53Calib)
  [Md32IsTargetPos] -> Subsystem1/34(Md32IsTargetPos)
  [Md53IsTargetPosZone] -> Subsystem1/39(Md53IsTargetPosZone)
  [Md32IsTargetPosAlready] -> Subsystem1/36(Md32IsTargetPosAlready)
  [Md53IsTargetPosAlready] -> Subsystem1/37(Md53IsTargetPosAlready)
  [Md53IsTargetPos] -> Subsystem1/35(Md53IsTargetPos)
  [Md32IsTargetPosZone] -> Subsystem1/38(Md32IsTargetPosZone)
  Md8R2RBkReclnUpwdDnwdTrgtPosCalib_TrgtPosArray_read/1 -> [Md8Calib]
  Md9R2RBkReclnUpwdDnwdTrgtPosCalib_TrgtPosArray_read/1 -> [Md9Calib]
  Md56R2RBkReclnUpwdDnwdTrgtPosCalib_TrgtPosArray_read/1 -> [Md56Calib]
  [PosDelta] -> Subsystem14/4(Delta)
  Subsystem14/2(IsPosZone) -> [Md8IsTargetPosZone]
  [PosV] -> Subsystem14/1(PosV)
  Subsystem14/1(IsPos) -> [Md8IsTargetPos]
  Subsystem14/3(IsPosAlready) -> [Md8IsTargetPosAlready]
  [Pos] -> Subsystem14/2(Pos)
  [Md8Calib] -> Subsystem14/3(CalibArray)
  [PosTolr] -> Subsystem14/5(Tolr)
  [PosTolr] -> Subsystem15/5(Tolr)
  [Md9Calib] -> Subsystem15/3(CalibArray)
  [Pos] -> Subsystem15/2(Pos)
  Subsystem15/3(IsPosAlready) -> [Md9IsTargetPosAlready]
  Subsystem15/1(IsPos) -> [Md9IsTargetPos]
  [PosV] -> Subsystem15/1(PosV)
  Subsystem15/2(IsPosZone) -> [Md9IsTargetPosZone]
  [PosDelta] -> Subsystem15/4(Delta)
  [PosDelta] -> Subsystem16/4(Delta)
  Subsystem16/2(IsPosZone) -> [Md56IsTargetPosZone]
  [PosV] -> Subsystem16/1(PosV)
  Subsystem16/1(IsPos) -> [Md56IsTargetPos]
  Subsystem16/3(IsPosAlready) -> [Md56IsTargetPosAlready]
  [Pos] -> Subsystem16/2(Pos)
  [Md56Calib] -> Subsystem16/3(CalibArray)
  [PosTolr] -> Subsystem16/5(Tolr)
  [Md8Calib] -> Subsystem/14(Md8Calib)
  [Md9Calib] -> Subsystem/15(Md9Calib)
  [Md56Calib] -> Subsystem/16(Md56Calib)
  [Md8IsTargetPos] -> Subsystem1/40(Md8IsTargetPos)
  [Md9IsTargetPos] -> Subsystem1/41(Md9IsTargetPos)
  [Md8IsTargetPosAlready] -> Subsystem1/43(Md8IsTargetPosAlready)
  [Md56IsTargetPos] -> Subsystem1/42(Md56IsTargetPos)
  [Md9IsTargetPosAlready] -> Subsystem1/44(Md9IsTargetPosAlready)
  [Md56IsTargetPosAlready] -> Subsystem1/45(Md56IsTargetPosAlready)
  [Md8IsTargetPosZone] -> Subsystem1/46(Md8IsTargetPosZone)
  [Md9IsTargetPosZone] -> Subsystem1/47(Md9IsTargetPosZone)
  [Md56IsTargetPosZone] -> Subsystem1/48(Md56IsTargetPosZone)
  Switch/1 -> MdXXSecRwRtStBkReclnEnIsTargetPosAlready_Val_write/1
  Data Type Conversion2/1 -> Switch/3, Bitwise Operator/1
  Bitwise Operator/1 -> Switch/1
  IfVeSMSbSecRwRtStCshnFrntUpwdDnwdMovConfig_Val_read/1 -> Switch/2
  Constant/1 -> Bitwise Operator1/1
  Bitwise Operator1/1 -> Bitwise Operator/2
  Md58R2RBkReclnUpwdDnwdTrgtPosCalib_TrgtPosArray_read/1 -> [Md58Calib]
  Md57R2RBkReclnUpwdDnwdTrgtPosCalib_TrgtPosArray_read/1 -> [Md57Calib]
  [PosTolr] -> Subsystem17/5(Tolr)
  [Md57Calib] -> Subsystem17/3(CalibArray)
  [Pos] -> Subsystem17/2(Pos)
  Subsystem17/3(IsPosAlready) -> [Md57IsTargetPosAlready]
  Subsystem17/1(IsPos) -> [Md57IsTargetPos]
  [PosV] -> Subsystem17/1(PosV)
  Subsystem17/2(IsPosZone) -> [Md57IsTargetPosZone]
  [PosDelta] -> Subsystem17/4(Delta)
  [PosDelta] -> Subsystem18/4(Delta)
  Subsystem18/2(IsPosZone) -> [Md58IsTargetPosZone]
  [PosV] -> Subsystem18/1(PosV)
  Subsystem18/1(IsPos) -> [Md58IsTargetPos]
  Subsystem18/3(IsPosAlready) -> [Md58IsTargetPosAlready]
  [Pos] -> Subsystem18/2(Pos)
  [Md58Calib] -> Subsystem18/3(CalibArray)
  [PosTolr] -> Subsystem18/5(Tolr)
  [Md57Calib] -> Subsystem/17(Md57Calib)
  [Md58Calib] -> Subsystem/18(Md58Calib)
  [is7s] -> Subsystem/19(is7s)
  Constant1/1 -> Bitwise Operator2/1
  Bitwise Operator2/1 -> Bitwise Operator/3
  Md62SecRwRtStBkReclnTrgtPosCalib_TrgtPosArray_read/1 -> [Md62Calib]
  Md61SecRwRtStBkReclnTrgtPosCalib_TrgtPosArray_read/1 -> [Md61Calib]
  [PosTolr] -> Subsystem19/5(Tolr)
  [Md61Calib] -> Subsystem19/3(CalibArray)
  [Pos] -> Subsystem19/2(Pos)
  Subsystem19/3(IsPosAlready) -> [Md61IsTargetPosAlready]
  Subsystem19/1(IsPos) -> [Md61IsTargetPos]
  [PosV] -> Subsystem19/1(PosV)
  Subsystem19/2(IsPosZone) -> [Md61IsTargetPosZone]
  [PosDelta] -> Subsystem19/4(Delta)
  [PosDelta] -> Subsystem20/4(Delta)
  Subsystem20/2(IsPosZone) -> [Md62IsTargetPosZone]
  [PosV] -> Subsystem20/1(PosV)
  Subsystem20/1(IsPos) -> [Md62IsTargetPos]
  Subsystem20/3(IsPosAlready) -> [Md62IsTargetPosAlready]
  [Pos] -> Subsystem20/2(Pos)
  [Md62Calib] -> Subsystem20/3(CalibArray)
  [PosTolr] -> Subsystem20/5(Tolr)
  [Md61Calib] -> Subsystem/20(Md61Calib)
  [Md62Calib] -> Subsystem/21(Md62Calib)
  [Md61IsTargetPos] -> Subsystem1/49(Md61IsTargetPos)
  [Md62IsTargetPos] -> Subsystem1/50(Md62IsTargetPos)
  [Md61IsTargetPosAlready] -> Subsystem1/51(Md61IsTargetPosAlready)
  [Md62IsTargetPosAlready] -> Subsystem1/52(Md62IsTargetPosAlready)
  [Md61IsTargetPosZone] -> Subsystem1/53(Md61IsTargetPosZone)
  [Md62IsTargetPosZone] -> Subsystem1/54(Md62IsTargetPosZone)
  Md28R2RBkReclnUpwdDnwdTrgtPosCalib_TrgtPosArray_read/1 -> [Md15Calib]
  VIPExitRR2RBkReclnUpwdDnwdTrgtPosCalib_TrgtPosArray_read/1 -> [Md28Calib]

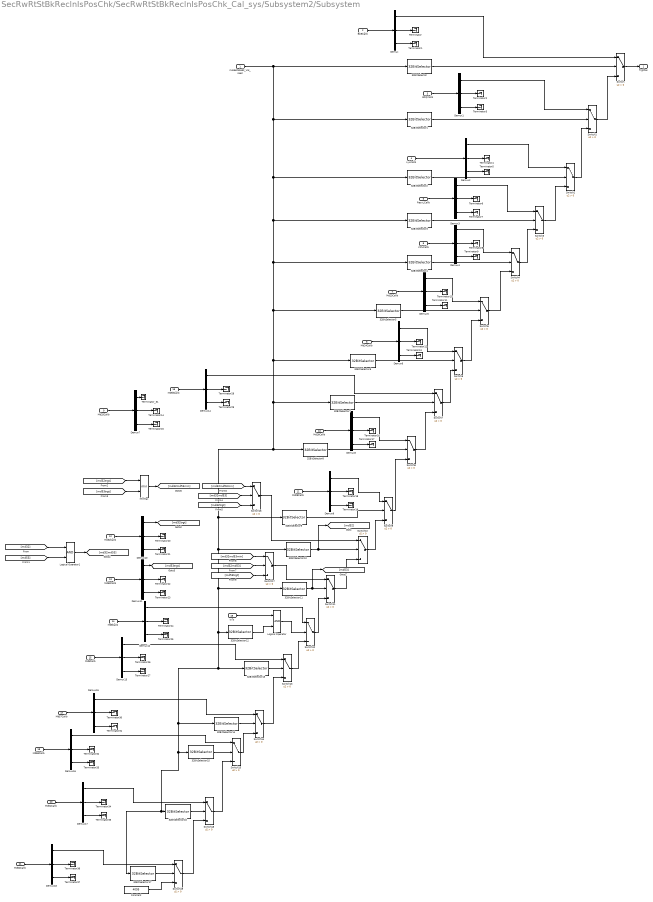
== system SecRwRtStBkReclnIsPosChk/SecRwRtStBkReclnIsPosChk_Cal_sys/Subsystem2/Subsystem ==
  modestate32_Val_read : Inport
  EZECalib : Inport  Port=2
  EZQCalib : Inport  Port=3
  LyLCalib : Inport  Port=4
  RecvLCalib : Inport  Port=5
  VIPLCalib : Inport  Port=6
  Md23Calib : Inport  Port=7
  Md24Calib : Inport  Port=8
  Md25Calib : Inport  Port=9
  Md26Calib : Inport  Port=10
  Md28Calib : Inport  Port=11
  Md32Calib : Inport  Port=12
  Md53Calib : Inport  Port=13
  Md8Calib : Inport  Port=14
  Md9Calib : Inport  Port=15
  Md56Calib : Inport  Port=16
  Md57Calib : Inport  Port=17
  Md58Calib : Inport  Port=18
  is7s : Inport  Port=19
  Md61Calib : Inport  Port=20
  Md62Calib : Inport  Port=21
  32BitSelector : StIsPosChkLib/32BitSelector  BitNum=0
  32BitSelector1 : StIsPosChkLib/32BitSelector  BitNum=3
  32BitSelector10 : StIsPosChkLib/32BitSelector  BitNum=31
  32BitSelector11 : StIsPosChkLib/32BitSelector  BitNum=17
  32BitSelector12 : StIsPosChkLib/32BitSelector  BitNum=7
  32BitSelector13 : StIsPosChkLib/32BitSelector  BitNum=8
  32BitSelector14 : StIsPosChkLib/32BitSelector  BitNum=20
  32BitSelector15 : StIsPosChkLib/32BitSelector  BitNum=21
  32BitSelector16 : StIsPosChkLib/32BitSelector  BitNum=5
  32BitSelector17 : StIsPosChkLib/32BitSelector  BitNum=6
  32BitSelector2 : StIsPosChkLib/32BitSelector  BitNum=14
  32BitSelector3 : StIsPosChkLib/32BitSelector  BitNum=12
  32BitSelector4 : StIsPosChkLib/32BitSelector  BitNum=11
  32BitSelector5 : StIsPosChkLib/32BitSelector  BitNum=22
  32BitSelector6 : StIsPosChkLib/32BitSelector  BitNum=23
  32BitSelector7 : StIsPosChkLib/32BitSelector  BitNum=24
  32BitSelector8 : StIsPosChkLib/32BitSelector  BitNum=25
  32BitSelector9 : StIsPosChkLib/32BitSelector  BitNum=27
  Constant : Constant  Value=4095  OutDataTypeStr=uint16
  Demux{,1..18} (19 alike) : Demux  Outputs=3
  Logical Operator : Logic  AllPortsSameDT=off  OutDataTypeStr=boolean
  Logical Operator1 : Logic  AllPortsSameDT=off  OutDataTypeStr=boolean
  MinMax : MinMax  Inputs=2
  Switch{,1..19} (20 alike) : Switch  Criteria=u2 > Threshold  SaturateOnIntegerOverflow=off  InputSameDT=off
  Terminator{,1..37} (38 alike) : Terminator
  Terminator_31 : Terminator
  TrgtPos : Outport  VectorParamsAs1DForOutWhenUnconnected=off
      settings: EnsureOutportIsVirtual=on
  wires:
  32BitSelector/1 -> Switch/2
  Demux/1 -> Switch/1
  Demux/3 -> Terminator1/1
  Demux/2 -> Terminator/1
  EZECalib/1 -> Demux/1
  EZQCalib/1 -> Demux1/1
  Demux1/2 -> Terminator2/1
  Demux1/3 -> Terminator3/1
  Demux1/1 -> Switch1/1
  Switch/1 -> TrgtPos/1
  Switch1/1 -> Switch/3
  32BitSelector1/1 -> Switch1/2
  Switch2/1 -> Switch1/3
  Switch3/1 -> Switch2/3
  Switch4/1 -> Switch3/3
  32BitSelector2/1 -> Switch2/2
  32BitSelector3/1 -> Switch3/2
  32BitSelector4/1 -> Switch4/2
  RecvLCalib/1 -> Demux3/1
  Demux3/2 -> Terminator6/1
  Demux3/3 -> Terminator7/1
  Demux3/1 -> Switch3/1
  Demux4/1 -> Switch4/1
  Demux4/3 -> Terminator9/1
  Demux4/2 -> Terminator8/1
  VIPLCalib/1 -> Demux4/1
  Md23Calib/1 -> Demux5/1
  Demux5/2 -> Terminator10/1
  Demux5/3 -> Terminator11/1
  Demux5/1 -> Switch5/1
  32BitSelector5/1 -> Switch5/2
  Switch5/1 -> Switch4/3
  Switch6/1 -> Switch5/3
  32BitSelector6/1 -> Switch6/2
  Demux6/1 -> Switch6/1
  Demux6/3 -> Terminator13/1
  Demux6/2 -> Terminator12/1
  Md24Calib/1 -> Demux6/1
  Md25Calib/1 -> Demux7/1
  Demux7/2 -> Terminator14/1
  Demux7/3 -> Terminator15/1
  32BitSelector7/1 -> Switch7/2
  Switch7/1 -> Switch6/3
  Switch8/1 -> Switch7/3
  32BitSelector8/1 -> Switch8/2
  Demux8/1 -> Switch8/1
  Demux8/3 -> Terminator17/1
  Demux8/2 -> Terminator16/1
  Md26Calib/1 -> Demux8/1
  Switch9/1 -> Switch8/3
  Demux9/3 -> Terminator19/1
  Demux9/2 -> Terminator18/1
  Md28Calib/1 -> Demux9/1
  32BitSelector9/1 -> Switch9/2
  Demux9/1 -> Switch9/1
  modestate32_Val_read/1 -> 32BitSelector/1, 32BitSelector1/1, 32BitSelector2/1, 32BitSelector3/1, 32BitSelector9/1, 32BitSelector10/1, 32BitSelector14/1, 32BitSelector17/1, 32BitSelector16/1, 32BitSelector15/1, 32BitSelector13/1, 32BitSelector12/1, 32BitSelector11/1, 32BitSelector8/1, 32BitSelector7/1, 32BitSelector6/1, 32BitSelector5/1, 32BitSelector4/1
  Switch10/1 -> Switch9/3
  Switch11/1 -> Switch10/3
  32BitSelector10/1 -> [md32], Switch10/2
  32BitSelector11/1 -> [md53], Switch11/2
  Demux10/1 -> [md32trgt]
  Demux10/2 -> Terminator20/1
  Demux10/3 -> Terminator21/1
  Md32Calib/1 -> Demux10/1
  Demux11/1 -> [md53trgt]
  Demux11/2 -> Terminator22/1
  Demux11/3 -> Terminator23/1
  Md53Calib/1 -> Demux11/1
  Md8Calib/1 -> Demux12/1
  Demux12/3 -> Terminator25/1
  Demux12/2 -> Terminator24/1
  Demux12/1 -> Switch12/1
  Switch12/1 -> Switch11/3
  Switch13/1 -> Switch12/3
  32BitSelector13/1 -> Switch13/2
  Demux13/1 -> Switch13/1
  Demux13/2 -> Terminator26/1
  Demux13/3 -> Terminator27/1
  Md9Calib/1 -> Demux13/1
  Md56Calib/1 -> Demux14/1
  Demux14/3 -> Terminator29/1
  Demux14/2 -> Terminator28/1
  Demux14/1 -> Switch7/1
  Demux7/1 -> Terminator_31/1
  Switch14/1 -> Switch13/3
  Switch15/1 -> Switch14/3
  32BitSelector14/1 -> Switch14/2
  32BitSelector15/1 -> Switch15/2
  Md57Calib/1 -> Demux15/1
  Demux15/3 -> Terminator31/1
  Demux15/2 -> Terminator30/1
  Demux15/1 -> Switch14/1
  Demux16/1 -> Switch15/1
  Demux16/2 -> Terminator32/1
  Demux16/3 -> Terminator33/1
  Md58Calib/1 -> Demux16/1
  is7s/1 -> Logical Operator/1
  32BitSelector12/1 -> Logical Operator/2
  Logical Operator/1 -> Switch12/2
  [md32] -> Logical Operator1/1
  [md53] -> Logical Operator1/2
  [md32trgt] -> MinMax/1
  [md53trgt] -> MinMax/2
  Logical Operator1/1 -> [md32md53]
  [md32md53] -> Switch16/2
  [md32trgt] -> Switch16/3
  Switch16/1 -> Switch10/1
  MinMax/1 -> [md32md53min]
  [md32md53min] -> Switch16/1
  Switch17/1 -> Switch11/1
  [md32md53] -> Switch17/2
  [md32md53min] -> Switch17/1
  [md53trgt] -> Switch17/3
  Switch18/1 -> Switch15/3
  Switch19/1 -> Switch18/3
  Constant/1 -> Switch19/3
  32BitSelector16/1 -> Switch18/2
  32BitSelector17/1 -> Switch19/2
  Md61Calib/1 -> Demux17/1
  Demux17/3 -> Terminator35/1
  Demux17/2 -> Terminator34/1
  Demux17/1 -> Switch18/1
  Demux18/1 -> Switch19/1
  Demux18/2 -> Terminator36/1
  Demux18/3 -> Terminator37/1
  Md62Calib/1 -> Demux18/1
  Demux2/2 -> Terminator4/1
  Demux2/3 -> Terminator5/1
  LyLCalib/1 -> Demux2/1
  Demux2/1 -> Switch2/1
